simulink model "APP_DD21"  (R2016b)
settings: configuration reference "CodeGenConfigSet" (kept outside this file)
values from neighbouring files (symbols this model uses):
  APP_tiSRCHighDefDeb_C = Calibration.Parameter    [init_APP_DD2.m]
  APP_tiSRCHighOKDeb_C = Calibration.Parameter    [init_APP_DD2.m]
  APP_tiSRCLowDefDeb_C = Calibration.Parameter    [init_APP_DD2.m]
  APP_tiSRCLowOKDeb_C = Calibration.Parameter    [init_APP_DD2.m]
  APP_uRaw2Def_C = Calibration.Parameter    [init_APP_DD2.m]
  APP_uRaw2SRCHigh_C = Calibration.Parameter    [init_APP_DD2.m]
  APP_uRaw2SRCLow_C = Calibration.Parameter    [init_APP_DD2.m]
undefined symbols (not defined in the file or in its folder): APP_DD2_DT
libraries: CXLib x6
settings Model: Creator=lenovo  LastModifiedBy=lenovo
settings ConfigSetRef: SourceLocation=Base Workspace

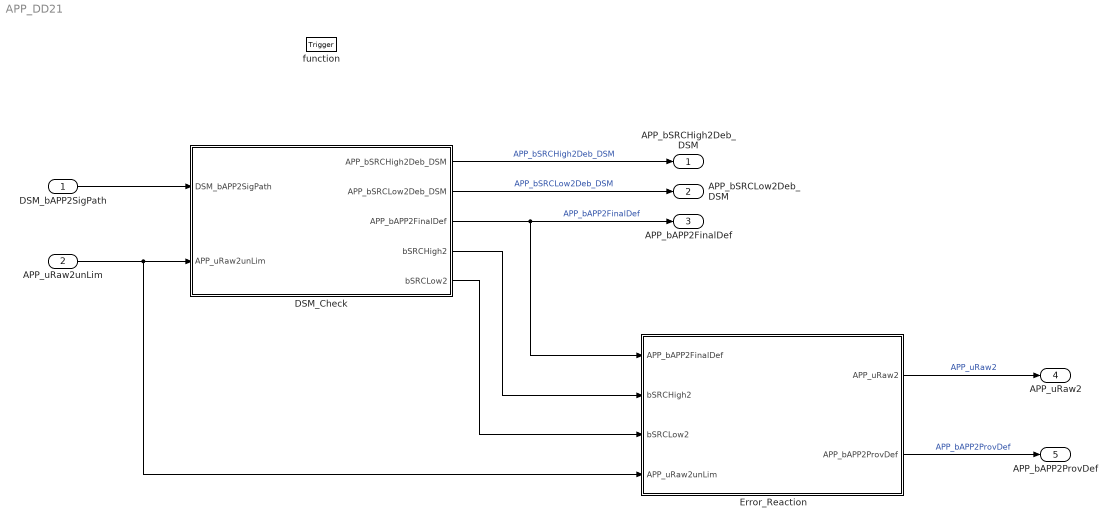
== system APP_DD21 ==
  DSM_bAPP2SigPath : Inport  Description=status of FId_APP2SigPath  OutMin=0  OutMax=1  OutDataTypeStr=boolean
  APP_uRaw2unLim : Inport  Tag=mv  Description=Acceleration pedal sensor 2 unlimited raw value  Port=2  OutMin=0  OutMax=5000  OutDataTypeStr=Ad_mv
  function : TriggerPort  TriggerType=function-call  VariantControl=Variant
  DSM_Check : Subsystem
  Error_Reaction : Subsystem
  APP_bSRCHigh2Deb_DSM : Outport  Description=Status debounced SRC-High error Sensor 2  OutMin=0  OutMax=1  OutDataTypeStr=boolean
  APP_bSRCLow2Deb_DSM : Outport  Description=Status debounced SRC-Low error Sensor 2  Port=2  OutMin=0  OutMax=1  OutDataTypeStr=boolean
  APP_bAPP2FinalDef : Outport  Description=Status Sensor 2 of the acceleration pedal finally defect  Port=3  OutMin=0  OutMax=1  OutDataTypeStr=boolean
  APP_uRaw2 : Outport  Tag=mv  Description=Acceleration Pedal Position E  Port=4  OutMin=0  OutMax=5000  OutDataTypeStr=Ad_mv
  APP_bAPP2ProvDef : Outport  Description=Status Sensor 2 of the acceleration pedal temporary defect  Port=5  OutMin=0  OutMax=1  OutDataTypeStr=boolean
  wires:
  DSM_Check/3(APP_bAPP2FinalDef) -> APP_bAPP2FinalDef/1, Error_Reaction/1(APP_bAPP2FinalDef)  "APP_bAPP2FinalDef"
  APP_uRaw2unLim/1 -> Error_Reaction/4(APP_uRaw2unLim), DSM_Check/2(APP_uRaw2unLim)
  DSM_bAPP2SigPath/1 -> DSM_Check/1(DSM_bAPP2SigPath)
  DSM_Check/1(APP_bSRCHigh2Deb_DSM) -> APP_bSRCHigh2Deb_DSM/1  "APP_bSRCHigh2Deb_DSM"
  DSM_Check/2(APP_bSRCLow2Deb_DSM) -> APP_bSRCLow2Deb_DSM/1  "APP_bSRCLow2Deb_DSM"
  DSM_Check/4(bSRCHigh2) -> Error_Reaction/2(bSRCHigh2)
  DSM_Check/5(bSRCLow2) -> Error_Reaction/3(bSRCLow2)
  Error_Reaction/1(APP_uRaw2) -> APP_uRaw2/1  "APP_uRaw2"
  Error_Reaction/2(APP_bAPP2ProvDef) -> APP_bAPP2ProvDef/1  "APP_bAPP2ProvDef"

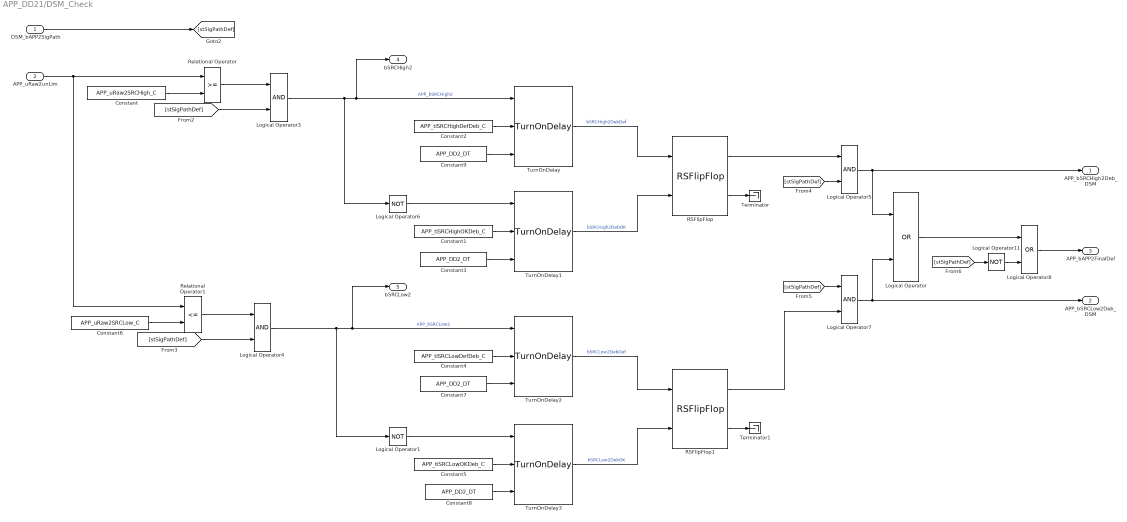
== system APP_DD21/DSM_Check ==
  DSM_bAPP2SigPath : Inport  Tag=-  Description=status of FId_APP1SigPath  OutMin=0  OutMax=1  OutDataTypeStr=boolean
  APP_uRaw2unLim : Inport  Tag=mv  Description=Acceleration pedal sensor 2 unlimited raw value  Port=2  OutMin=0  OutMax=5000  OutDataTypeStr=Ad_mv
  Constant : Constant  Value=APP_uRaw2SRCHigh_C
  Constant1 : Constant  Value=APP_tiSRCHighOKDeb_C
  Constant2 : Constant  Value=APP_tiSRCHighDefDeb_C
  Constant{3,7..9} (4 alike) : Constant  Value=APP_DD2_DT  OutDataTypeStr=Inherit: Inherit via back propagation
  Constant4 : Constant  Value=APP_tiSRCLowDefDeb_C
  Constant5 : Constant  Value=APP_tiSRCLowOKDeb_C
  Constant6 : Constant  Value=APP_uRaw2SRCLow_C
  Logical Operator : Logic  Operator=OR  AllPortsSameDT=off  OutDataTypeStr=boolean
  Logical Operator1 : Logic  Operator=NOT  AllPortsSameDT=off  OutDataTypeStr=boolean
  Logical Operator11 : Logic  Operator=NOT  AllPortsSameDT=off  OutDataTypeStr=boolean
  Logical Operator{3..5,7} (4 alike) : Logic  AllPortsSameDT=off  OutDataTypeStr=boolean
  Logical Operator6 : Logic  Operator=NOT  AllPortsSameDT=off  OutDataTypeStr=boolean
  Logical Operator8 : Logic  Operator=OR  AllPortsSameDT=off  OutDataTypeStr=boolean
  RSFlipFlop : CXLib/RSFlipFlop
  RSFlipFlop1 : CXLib/RSFlipFlop
  Relational Operator : RelationalOperator  OutDataTypeStr=boolean  RndMeth=Nearest  InputSameDT=on
  Relational Operator1 : RelationalOperator  Operator=<=  OutDataTypeStr=boolean  RndMeth=Nearest  InputSameDT=on
  Terminator : Terminator
  Terminator1 : Terminator
  TurnOnDelay{,1..3} (4 alike) : CXLib/TurnOnDelay
  APP_bSRCHigh2Deb_DSM : Outport  Tag=-  Description=Status debounced SRC-High error Sensor 1  OutMin=0  OutMax=1  OutDataTypeStr=boolean
  APP_bSRCLow2Deb_DSM : Outport  Tag=-  Description=Status debounced SRC-Low error Sensor 1  Port=2  OutMin=0  OutMax=1  OutDataTypeStr=boolean
  APP_bAPP2FinalDef : Outport  Tag=-  Description=Status Sensor 2 of the acceleration pedal finally defect  Port=3  OutMin=0  OutMax=1  OutDataTypeStr=boolean
  bSRCHigh2 : Outport  Port=4
  bSRCLow2 : Outport  Port=5
  wires:
  Logical Operator8/1 -> APP_bAPP2FinalDef/1
  Logical Operator11/1 -> Logical Operator8/2
  [stSigPathDef] -> Logical Operator5/2
  Relational Operator/1 -> Logical Operator3/1
  DSM_bAPP2SigPath/1 -> [stSigPathDef]
  Constant6/1 -> Relational Operator1/2
  [stSigPathDef] -> Logical Operator3/2
  Constant/1 -> Relational Operator/2
  [stSigPathDef] -> Logical Operator7/1
  APP_uRaw2unLim/1 -> Relational Operator/1, Relational Operator1/1
  Logical Operator4/1 -> bSRCLow2/1, TurnOnDelay2/1, Logical Operator1/1  "APP_bSRCLow2"
  Logical Operator3/1 -> bSRCHigh2/1, TurnOnDelay/1, Logical Operator6/1  "APP_bSRCHigh2"
  Logical Operator7/1 -> APP_bSRCLow2Deb_DSM/1, Logical Operator/2
  Relational Operator1/1 -> Logical Operator4/1
  [stSigPathDef] -> Logical Operator4/2
  Logical Operator5/1 -> APP_bSRCHigh2Deb_DSM/1, Logical Operator/1
  [stSigPathDef] -> Logical Operator11/1
  Logical Operator/1 -> Logical Operator8/1
  Constant8/1 -> TurnOnDelay3/3
  Constant7/1 -> TurnOnDelay2/3
  Constant3/1 -> TurnOnDelay1/3
  Constant9/1 -> TurnOnDelay/3
  RSFlipFlop/2 -> Terminator/1
  RSFlipFlop1/2 -> Terminator1/1
  Constant2/1 -> TurnOnDelay/2
  TurnOnDelay/1 -> RSFlipFlop/1  "bSRCHigh2DebDef"
  Logical Operator6/1 -> TurnOnDelay1/1
  Constant5/1 -> TurnOnDelay3/2
  TurnOnDelay3/1 -> RSFlipFlop1/2  "bSRCLow2DebOK"
  Constant4/1 -> TurnOnDelay2/2
  TurnOnDelay1/1 -> RSFlipFlop/2  "bSRCHigh2DebOK"
  Logical Operator1/1 -> TurnOnDelay3/1
  RSFlipFlop/1 -> Logical Operator5/1
  TurnOnDelay2/1 -> RSFlipFlop1/1  "bSRCLow2DebDef"
  Constant1/1 -> TurnOnDelay1/2
  RSFlipFlop1/1 -> Logical Operator7/2

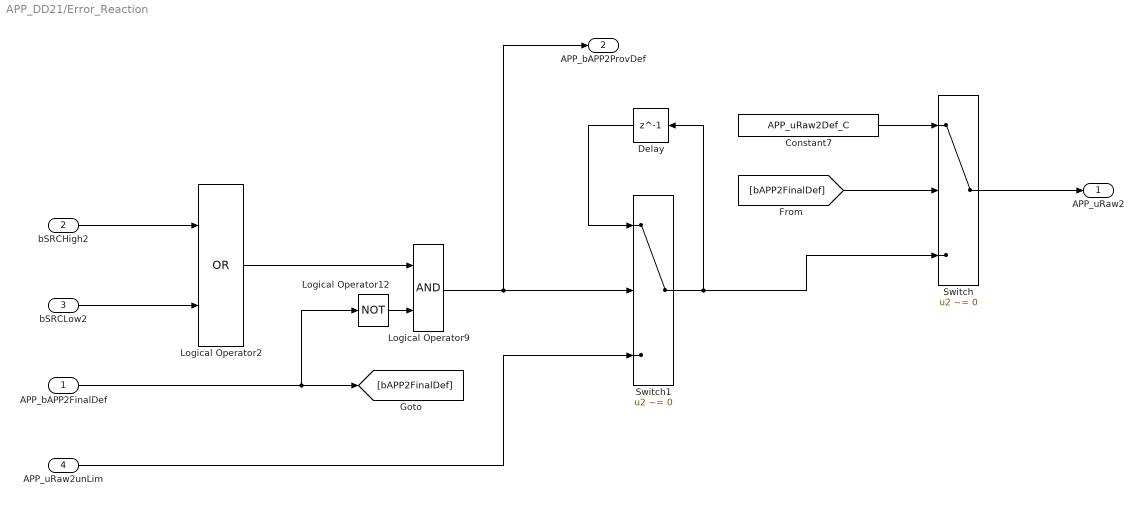
== system APP_DD21/Error_Reaction ==
  APP_bAPP2FinalDef : Inport
  bSRCHigh2 : Inport  Port=2
  bSRCLow2 : Inport  Port=3
  APP_uRaw2unLim : Inport  Port=4
  Constant7 : Constant  Value=APP_uRaw2Def_C
  Delay : Delay  DelayLength=1  InitialCondition=0
  Logical Operator12 : Logic  Operator=NOT  AllPortsSameDT=off  OutDataTypeStr=boolean
  Logical Operator2 : Logic  Operator=OR  AllPortsSameDT=off  OutDataTypeStr=boolean
  Logical Operator9 : Logic  AllPortsSameDT=off  OutDataTypeStr=boolean
  Switch : Switch  Criteria=u2 ~= 0
  Switch1 : Switch  Criteria=u2 ~= 0
  APP_uRaw2 : Outport  Tag=mv  Description=Acceleration Pedal Position E  OutMin=0  OutMax=5000  OutDataTypeStr=Ad_mv
  APP_bAPP2ProvDef : Outport  Tag=-  Description=Status Sensor 2 of the acceleration pedal temporary defect  Port=2  OutMin=0  OutMax=1  OutDataTypeStr=boolean
  wires:
  Constant7/1 -> Switch/1
  Logical Operator2/1 -> Logical Operator9/1
  Logical Operator12/1 -> Logical Operator9/2
  Logical Operator9/1 -> APP_bAPP2ProvDef/1, Switch1/2
  Switch/1 -> APP_uRaw2/1
  Switch1/1 -> Delay/1, Switch/3
  APP_bAPP2FinalDef/1 -> [bAPP2FinalDef], Logical Operator12/1
  Delay/1 -> Switch1/1
  APP_uRaw2unLim/1 -> Switch1/3
  bSRCLow2/1 -> Logical Operator2/2
  bSRCHigh2/1 -> Logical Operator2/1
  [bAPP2FinalDef] -> Switch/2
